simulink model "Realization_of_Filter"  (R2020a)
settings: Solver=VariableStepAuto  StartTime=0.0  StopTime=10.0  RelTol=1e-3
PreLoadFcn:
  | def fun1:
  |   Gain_1=0.4
  |   Gain_2=0.5
  |   Gain_3=0.25
model workspace (MAT data in the model file):
  Gain_1 = 0.4
  Gain_2 = 0.5
  Gain_3 = 0.25
settings Model: Creator=INDRAJIT MARATHE  LastModifiedBy=INDRAJIT MARATHE

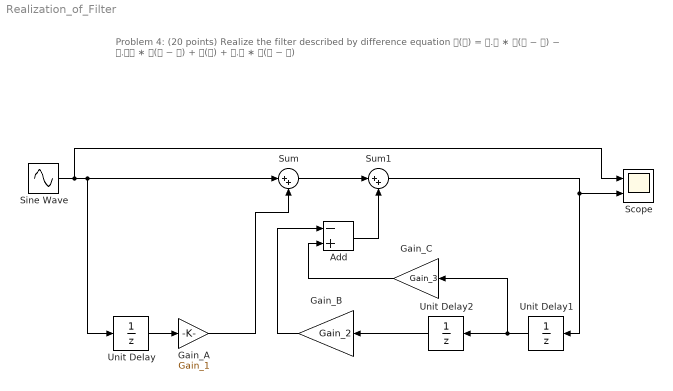
== system Realization_of_Filter ==
  note: Problem 4: (20 points)
      | Realize the filter described by difference equation
      |  𝐲(𝐧) = 𝟎.𝟓 ∗ 𝐲(𝐧 − 𝟏) − 𝟎.𝟐𝟓 ∗ 𝐲(𝐧 − 𝟐) + 𝐱(𝐧) + 𝟎.𝟒 ∗ 𝐱(𝐧 − 𝟏)
  Add : Sum  Inputs=-+
  Gain_A : Gain  Gain=Gain_1
  Gain_B : Gain  Gain=Gain_2
  Gain_C : Gain  Gain=Gain_3
  Scope : Scope  NumInputPorts=2
  Sine Wave : Sin  SampleTime=0
  Sum : Sum  Inputs=|++
  Sum1 : Sum  Inputs=|++
  Unit Delay : UnitDelay  SampleTime=-1  HasFrameUpgradeWarning=on
  Unit Delay1 : UnitDelay  SampleTime=-1  HasFrameUpgradeWarning=on
  Unit Delay2 : UnitDelay  SampleTime=-1  HasFrameUpgradeWarning=on
  wires:
  Unit Delay/1 -> Gain_A/1
  Sine Wave/1 -> Scope/1, Unit Delay/1, Sum/1
  Gain_A/1 -> Sum/2
  Unit Delay2/1 -> Gain_B/1
  Gain_B/1 -> Add/1
  Unit Delay1/1 -> Gain_C/1, Unit Delay2/1
  Gain_C/1 -> Add/2
  Sum1/1 -> Scope/2, Unit Delay1/1
  Sum/1 -> Sum1/1
  Add/1 -> Sum1/2
